simulink subsystem "CellMonitoringUnit"  (R2022a)
settings: Solver=VariableStepAuto  StartTime=0.0  StopTime=10.0  RelTol=1e-3
libraries: nesl_utility x6, fl_lib x6
settings Model: Creator=tshintai  LastModifiedBy=tshintai
settings DebuggingCC: UnconnectedInputMsg=warning  UnconnectedOutputMsg=warning  UnconnectedLineMsg=warning
settings RTWCC: DLArmComputeVersion=19.05

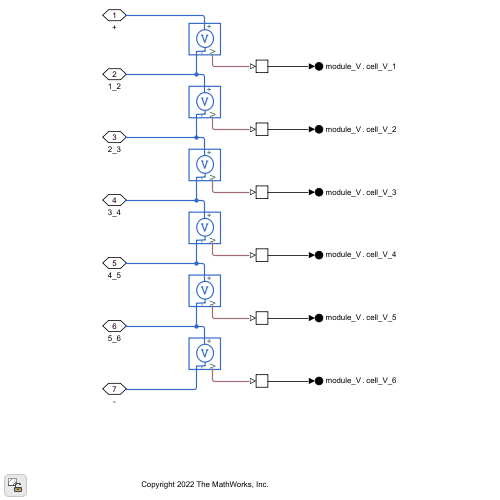
[thumbnail: Simulink's stored preview of the top-level diagram]
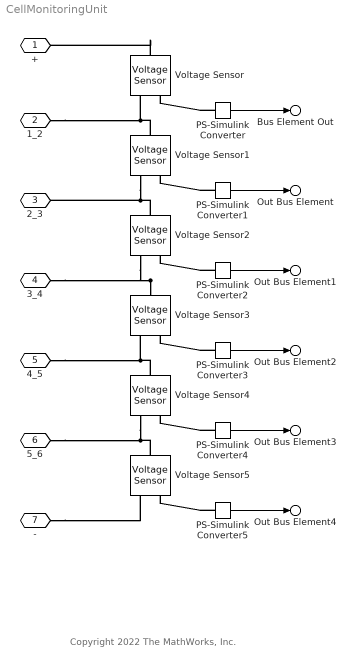
== system CellMonitoringUnit ==
  note: Copyright 2022 The MathWorks, Inc.
  PS-Simulink Converter{,1..5} (6 alike) : nesl_utility/PS-Simulink Converter  PhysicalDomain=network_engine_domain  SubClassName=ps_output  LeftPortType=input  RightPortType=output  PseudoPeriodic=off  Frequencies=[]  VectorFormat=1-D array  Unit=inherit  AffineConversion=off
      settings: SourceProductBaseCode=SS,PW,VE
  Voltage Sensor{,1..5} (6 alike) : fl_lib/Electrical/Electrical Sensors/Voltage Sensor
      settings: SourceProductBaseCode=PW,SS,VE
  + : PMIOPort  Side=Left
  1_2 : PMIOPort  Port=2  Side=Left
  2_3 : PMIOPort  Port=3  Side=Left
  3_4 : PMIOPort  Port=4  Side=Left
  4_5 : PMIOPort  Port=5  Side=Left
  5_6 : PMIOPort  Port=6  Side=Left
  - : PMIOPort  Port=7  Side=Left
  Bus Element Out : Outport  PortName=module_V  Element=cell_V_1
  Out Bus Element : Outport  PortName=module_V  Element=cell_V_2
  Out Bus Element1 : Outport  PortName=module_V  Element=cell_V_3
  Out Bus Element2 : Outport  PortName=module_V  Element=cell_V_4
  Out Bus Element3 : Outport  PortName=module_V  Element=cell_V_5
  Out Bus Element4 : Outport  PortName=module_V  Element=cell_V_6
  wires:
  PS-Simulink Converter5/1 -> Out Bus Element4/1
  PS-Simulink Converter4/1 -> Out Bus Element3/1
  PS-Simulink Converter3/1 -> Out Bus Element2/1
  PS-Simulink Converter2/1 -> Out Bus Element1/1
  PS-Simulink Converter1/1 -> Out Bus Element/1
  PS-Simulink Converter/1 -> Bus Element Out/1
  connections:
  Voltage Sensor3/LConn1 -- 3_4/RConn1 -- Voltage Sensor2/RConn2
  Voltage Sensor5/LConn1 -- Voltage Sensor4/RConn2 -- 5_6/RConn1
  Voltage Sensor4/LConn1 -- Voltage Sensor3/RConn2 -- 4_5/RConn1
  Voltage Sensor2/LConn1 -- 2_3/RConn1 -- Voltage Sensor1/RConn2
  Voltage Sensor1/LConn1 -- 1_2/RConn1 -- Voltage Sensor/RConn2
  PS-Simulink Converter5/LConn1 -- Voltage Sensor5/RConn1
  PS-Simulink Converter4/LConn1 -- Voltage Sensor4/RConn1
  PS-Simulink Converter3/LConn1 -- Voltage Sensor3/RConn1
  PS-Simulink Converter2/LConn1 -- Voltage Sensor2/RConn1
  PS-Simulink Converter1/LConn1 -- Voltage Sensor1/RConn1
  PS-Simulink Converter/LConn1 -- Voltage Sensor/RConn1
  -/RConn1 -- Voltage Sensor5/RConn2
  Voltage Sensor/LConn1 -- +/RConn1
